simulink model "Linefollow"  (R2023a)
settings: Solver=FixedStepDiscrete  StartTime=0.0  StopTime=15  FixedStep=0.01  RelTol=1e-3
undefined symbols (not defined in the file or in its folder): InputPWM, WheelSpeed
libraries: arduinolib x11, slpidlib x1, mobileRoboticsTrainingLib x1
settings Model: ExtModeTrigDuration=2  Creator=Boitumelo  LastModifiedBy=siyan
settings OptimizationCC: EnhancedBackFolding=on  PassReuseOutputArgsAs=Individual arguments  ZeroExternalMemoryAtStartup=off  ZeroInternalMemoryAtStartup=off  MaxStackSize=64  OptimizeBlockOrder=speed  DifferentSizesBufferReuse=on  OptimizationCustomize=off  EfficientTunableParamExpr=on
settings DebuggingCC: ParameterTunabilityLossMsg=error  UnconnectedInputMsg=warning  UnconnectedOutputMsg=warning  UnconnectedLineMsg=warning
settings HardwareCC: ProdBitPerPointer=32  ProdBitPerSizeT=32  ProdBitPerPtrDiffT=32  ProdLargestAtomicInteger=Long  ProdLargestAtomicFloat=Double  ProdWordSize=32  ProdHWDeviceType=ARM Compatible->ARM Cortex  UseEmbeddedCoderFeatures=off
settings ModelReferenceCC: EnableRefExpFcnMdlSchedulingChecks=on
settings SFSimCC: MATLABDynamicMemAlloc=off
settings RTWCC: Description=Embedded Coder  SystemTargetFile=ert.tlc  HardwareBoard=Arduino Nano 33 IoT  TemplateMakefile=ert_default_tmf  Toolchain=Arduino ARM  BuildConfiguration=Faster Runs  DLArmComputeVersion=19.05
settings CodeAppCC: ForceParamTrailComments=on  IgnoreCustomStorageClasses=off  OperatorAnnotations=on  SimulinkDataObjDesc=on  SFDataObjDesc=on  InsertBlockDesc=on
settings ERTTargetCC: SupportContinuousTime=on  SupportNonInlinedSFcns=on  SupportVariableSizeSignals=on  ExtModeTransport=3  ExtModeStaticAlloc=on  ExtModeAutomaticAllocSize=off  ExtModeStaticAllocSize=8192  ExtModeMexFile=ext_xcp  ExtModeIntrfLevel=Level2 - Open

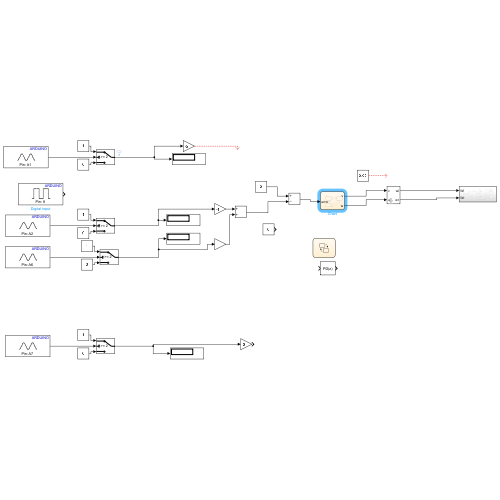
[thumbnail: Simulink's stored preview of the top-level diagram]
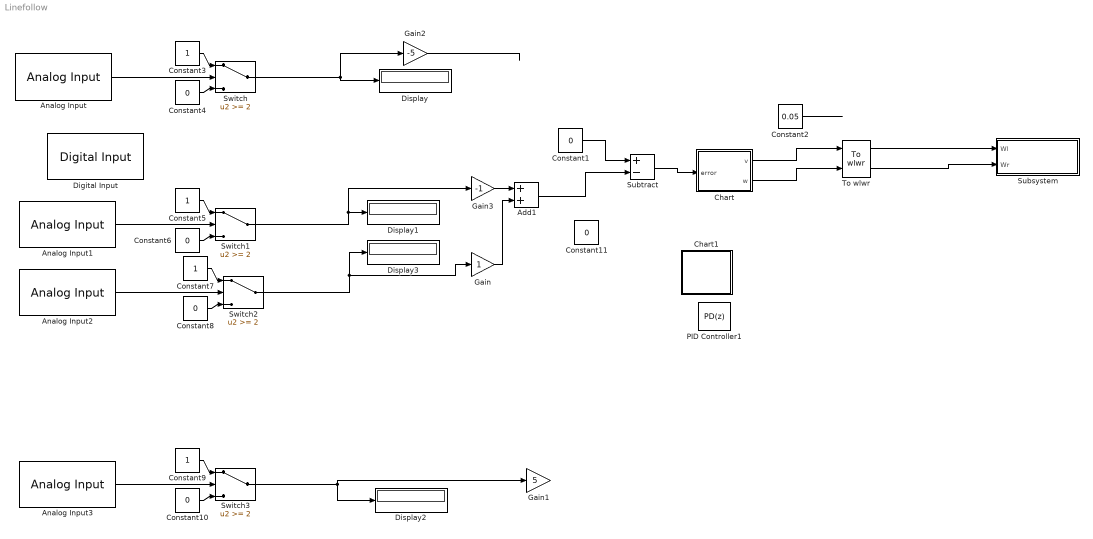
== system Linefollow ==
  Add1 : Sum
  Analog Input : arduinolib/Analog Input  pinNumber=1  ReadResultsOnly=off  ConversionTriggerSource=Software  ExternalTriggerType=uint32( 0 )  OutputDataType=uint16  EnableConversionCompleteNotify=off  EnableOuputStatus=off  SampleTime=-1  blockPlatform=arduino
  Analog Input1 : arduinolib/Analog Input  pinNumber=2  ReadResultsOnly=off  ConversionTriggerSource=Software  ExternalTriggerType=uint32( 0 )  OutputDataType=uint16  EnableConversionCompleteNotify=off  EnableOuputStatus=off  SampleTime=-1  blockPlatform=arduino
  Analog Input2 : arduinolib/Analog Input  pinNumber=6  ReadResultsOnly=off  ConversionTriggerSource=Software  ExternalTriggerType=uint32( 0 )  OutputDataType=uint16  EnableConversionCompleteNotify=off  EnableOuputStatus=off  SampleTime=-1  blockPlatform=arduino
  Analog Input3 : arduinolib/Analog Input  pinNumber=7  ReadResultsOnly=off  ConversionTriggerSource=Software  ExternalTriggerType=uint32( 0 )  OutputDataType=uint16  EnableConversionCompleteNotify=off  EnableOuputStatus=off  SampleTime=-1  blockPlatform=arduino
  Chart : Stateflow chart  TreatAsAtomicUnit=on
  Chart1 : Stateflow chart  TreatAsAtomicUnit=on
  Constant{1,4,6,8,10..11} (6 alike) : Constant  Value=0
  Constant2 : Constant  Value=0.05
  Constant{3,5,7,9} (4 alike) : Constant
  Digital Input : arduinolib/Digital Input  pinNumber=8  mode=Default  Direction=input  SampleTime=0.1  blockPlatform=arduino
  Display{,1..3} (4 alike) : Display
  Gain : Gain
  Gain1 : Gain  Gain=5
  Gain2 : Gain  Gain=-5
  Gain3 : Gain  Gain=-1
  PID Controller1 : slpidlib/PID Controller  Controller=PD  Form=Parallel  TimeDomain=Discrete-time  UseExternalTs=off  SampleTime=-1  IntegratorMethod=Forward Euler  FilterMethod=Forward Euler  ControllerParametersSource=internal  P=500  I=0  UseKiTs=off  D=0.01  N=100  UseFilter=on  TunerSelectOption=Transfer Function Based (PID Tuner App)  InitialConditionSource=internal  InitialConditionForIntegrator=0  InitialConditionForFilter=0  DifferentiatorICPrevScaledInput=0  ExternalReset=none  TrackingMode=off  Kt=1  LimitOutput=off  SatLimitsSource=internal  UpperSaturationLimit=0.32  LowerSaturationLimit=-0.32  LinearizeAsGain=on  AntiWindupMode=none  Kb=1  LimitIntegrator=off  UpperIntegratorSaturationLimit=inf  LowerIntegratorSaturationLimit=-inf  POutMin=[]  POutMax=[]  IOutMin=[]  IOutMax=[]  DOutMin=[]  DOutMax=[]  NOutMin=[]  NOutMax=[]  SumOutMin=[]  SumOutMax=[]  SaturationOutMin=[]  SaturationOutMax=[]  PParamMin=[]  PParamMax=[]  IParamMin=[]  IParamMax=[]  DParamMin=[]  DParamMax=[]  NParamMin=[]  NParamMax=[]  KbParamMin=[]  KbParamMax=[]  KtParamMin=[]  KtParamMax=[]  KbOutMin=[]  KbOutMax=[]  KtOutMin=[]  KtOutMax=[]  IntegratorOutMin=[]  IntegratorOutMax=[]  FilterOutMin=[]  FilterOutMax=[]  SumI1OutMin=[]  SumI1OutMax=[]  SumI2OutMin=[]  SumI2OutMax=[]  SumI3OutMin=[]  SumI3OutMax=[]  SumI4OutMin=[]  SumI4OutMax=[]  SumDOutMin=[]  SumDOutMax=[]  DifferentiatorOutMin=[]  DifferentiatorOutMax=[]  FilterDiffOutCoefMin=[]  FilterDiffOutCoefMax=[]  ReciprocalOutMin=[]  ReciprocalOutMax=[]  SumDenOutMin=[]  SumDenOutMax=[]  SumNumOutMin=[]  SumNumOutMax=[]  DivideOutMin=[]  DivideOutMax=[]  UdiffTsProdOutMin=[]  UdiffTsProdOutMax=[]  NTsProdOutMin=[]  NTsProdOutMax=[]  UintegralTsProdOutMin=[]  UintegralTsProdOutMax=[]  UngainTsProdOutMin=[]  UngainTsProdOutMax=[]  ClampingZeroOutDataTypeStr=Inherit: Inherit via back propagation  ClampingZeroOutMin=[]  ClampingZeroOutMax=[]  FilterDenConstantOutDataTypeStr=Inherit: Inherit via back propagation  FilterDenConstantOutMin=[]  FilterDenConstantOutMax=[]  PCopyOutDataTypeStr=Inherit: Inherit via back propagation  PCopyOutMin=[]  PCopyOutMax=[]  NCopyOutDataTypeStr=Inherit: Inherit via back propagation  NCopyOutMin=[]  NCopyOutMax=[]  IntegratorContinuousStateAttributes=''  IntegratorStateMustResolveToSignalObject=off  IntegratorRTWStateStorageClass=Auto  FilterContinuousStateAttributes=''  FilterStateMustResolveToSignalObject=off  FilterRTWStateStorageClass=Auto  ParallelPVariant=InternalParameters  IdealPVariant=Disabled  IVariant=Disabled  DVariant=InternalParameters  IntegratorVariant=Disabled  SatVariant=Disabled  AWVariant=Disabled  PCopyVariant=Disabled  TRVariant=Disabled  FdbkBlocksVariant=Forward  IdealPFdbkVariant=Disabled  SatFdbkVariant=Disabled  DerivativeFilterVariant=ForwardEulerFilter  NVariant=InternalParameters  NCopyVariant=Disabled  FilterICVariant=InternalICsFilter  IntegratorICVariant=Disabled  ExternalResetVariant=Disabled  TRSumVariant=Passthrough  SumFdbkVariant=Disabled  SumVariant=Sum_PD  TsampFilterVariant=InternalTs  TsampNgainVariant=Passthrough  TsampIntegralVariant=Disabled_SignalSpec  ExternalSaturationOutDataTypeStr=Inherit: Same as second input
  Subsystem : Subsystem
      settings: LibrarySourceBlock=|
      | hdlsllib/Ports &
      | Subsystems/Subsystem
  Subtract : Sum  Inputs=+-
  Switch{,1..3} (4 alike) : Switch  Threshold=2  SaturateOnIntegerOverflow=off  InputSameDT=off
  To wlwr : mobileRoboticsTrainingLib/To wlwr  axleLength=axleLength  wheelR=wheelR
      link override change parameters: Gain=[1 +axleLength/2; 1 -axleLength/2]
  wires:
  Switch3/1 -> Gain1/1, Display2/1
  Switch/1 -> Gain2/1, Display/1
  Switch1/1 -> Gain3/1, Display1/1
  Switch2/1 -> Display3/1, Gain/1
  Gain2/1 -> ?
  Constant1/1 -> Subtract/1
  Add1/1 -> Subtract/2
  Constant2/1 -> ?
  Subtract/1 -> Chart/1(error)
  Chart/2(w) -> To wlwr/2
  Gain3/1 -> Add1/1
  To wlwr/1 -> Subsystem/1(Wl)
  To wlwr/2 -> Subsystem/2(Wr)
  Analog Input/1 -> Switch/2
  Constant3/1 -> Switch/1
  Constant4/1 -> Switch/3
  Constant5/1 -> Switch1/1
  Constant6/1 -> Switch1/3
  Analog Input1/1 -> Switch1/2
  Constant7/1 -> Switch2/1
  Constant8/1 -> Switch2/3
  Analog Input2/1 -> Switch2/2
  Constant9/1 -> Switch3/1
  Constant10/1 -> Switch3/3
  Analog Input3/1 -> Switch3/2
  Gain/1 -> Add1/2
  Chart/1(v) -> To wlwr/1

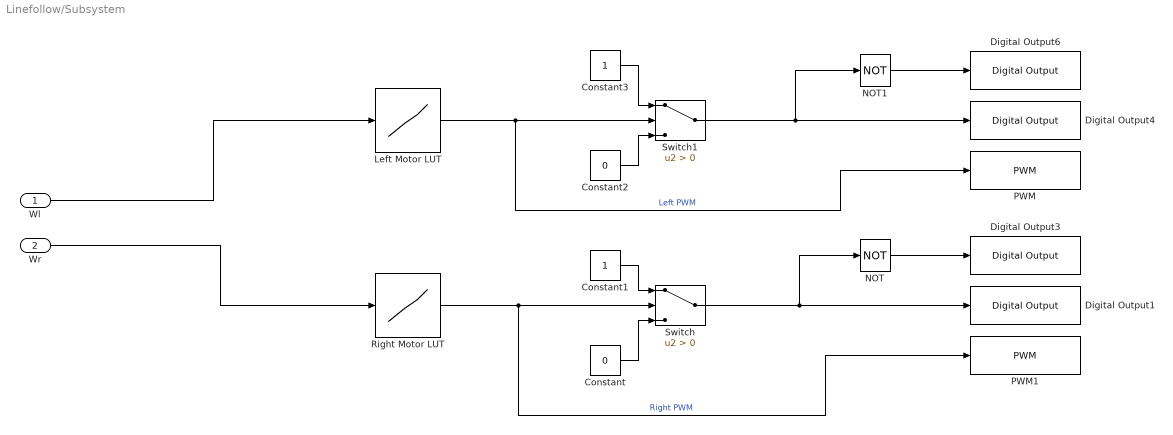
== system Linefollow/Subsystem ==
  Wl : Inport
  Wr : Inport  Port=2
  Constant : Constant  Value=0
  Constant1 : Constant
  Constant2 : Constant  Value=0
  Constant3 : Constant
  Digital Output1 : arduinolib/Digital Output  pinNumber=8  Direction=output  blockPlatform=arduino
  Digital Output3 : arduinolib/Digital Output  pinNumber=11  Direction=output  blockPlatform=arduino
  Digital Output4 : arduinolib/Digital Output  pinNumber=13  Direction=output  blockPlatform=arduino
  Digital Output6 : arduinolib/Digital Output  pinNumber=12  Direction=output  blockPlatform=arduino
  Left Motor LUT : Lookup_n-D  NumberOfTableDimensions=1  BreakpointsForDimension1=WheelSpeed  Table=InputPWM  InterpMethod=Nearest  ExtrapMethod=Clip  InternalRulePriority=Speed  RndMeth=Simplest
  NOT : Logic  Operator=NOT  IconShape=distinctive  AllPortsSameDT=off  OutDataTypeStr=boolean
  NOT1 : Logic  Operator=NOT  IconShape=distinctive  AllPortsSameDT=off  OutDataTypeStr=boolean
  PWM : arduinolib/PWM  pinNumber=9  frequencyType=Default  desiredFrequency=490.2  achievableFrequency=490.2
  PWM1 : arduinolib/PWM  pinNumber=10  frequencyType=Default  desiredFrequency=490.2  achievableFrequency=490.2
  Right Motor LUT : Lookup_n-D  NumberOfTableDimensions=1  BreakpointsForDimension1=WheelSpeed  Table=InputPWM  InterpMethod=Nearest  ExtrapMethod=Clip  InternalRulePriority=Speed  RndMeth=Simplest
  Switch : Switch  Criteria=u2 > Threshold  SaturateOnIntegerOverflow=off  InputSameDT=off
  Switch1 : Switch  Criteria=u2 > Threshold  SaturateOnIntegerOverflow=off  InputSameDT=off
  wires:
  Wr/1 -> Right Motor LUT/1
  Wl/1 -> Left Motor LUT/1
  Right Motor LUT/1 -> PWM1/1, Switch/2  "Right PWM"
  Left Motor LUT/1 -> PWM/1, Switch1/2  "Left PWM"
  NOT1/1 -> Digital Output6/1
  Constant1/1 -> Switch/1
  Constant/1 -> Switch/3
  Constant2/1 -> Switch1/3
  Constant3/1 -> Switch1/1
  Switch/1 -> NOT/1, Digital Output1/1
  Switch1/1 -> NOT1/1, Digital Output4/1
  NOT/1 -> Digital Output3/1

== stateflow chart Linefollow/Chart1 ==

== stateflow chart Linefollow/Chart ==
  state Straight
    entry:
    w =0
    v= 0.06
  state SteerRight
    entry:
    w = -1
    v=0.045
  state SteerLeft
    entry:
    w= 3.8
    v=0.045
  (default) -> Straight
  Straight -> SteerRight [order 1] : [error > 0.1]
  SteerRight -> Straight [order 1] : [error <0.1]
  Straight -> SteerLeft [order 2] : [error <-0.1]
  SteerLeft -> Straight [order 1] : [error >  -0.1]
  SteerLeft -> SteerRight [order 2] : [error>0.1]
  SteerRight -> SteerLeft [order 2] : [error < -0.1]
  data: v output; error input; w output
